simulink model "Test_Arithmetic_Operation_Bit_Comparator_Less_Than"  (Simulink 8.7)
settings: Solver=ode45  StartTime=0.0  StopTime=len  RelTol=1e-3
libraries: Arithmetic_Operations_Lib x1
settings Model: Creator=uzivatel  LastModifiedBy=Jozko Mrkvicka
settings DebuggingCC: SolverPrmCheckMsg=warning  StateNameClashWarn=warning

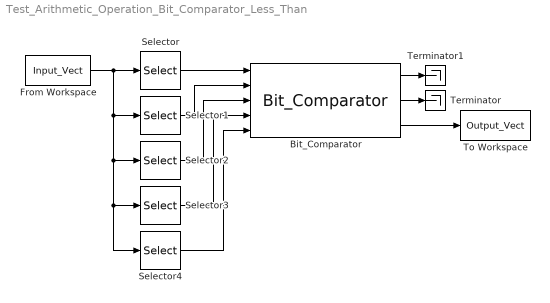
== system Test_Arithmetic_Operation_Bit_Comparator_Less_Than ==
  Bit_Comparator : Arithmetic_Operations_Lib/Arithmetic_Operations_Lib/Bit_Comparator
  From Workspace : FromWorkspace  VariableName=Input_Vect  SampleTime=1  Interpolate=off  OutputAfterFinalValue=Holding final value
  Selector : Selector  IndexMode=Zero-based  InputPortWidth=5  SampleTime=1  IndexOptions=Index vector (dialog)  Indices=0  OutputSizes=1
  Selector1 : Selector  IndexMode=Zero-based  InputPortWidth=5  SampleTime=1  IndexOptions=Index vector (dialog)  Indices=1  OutputSizes=1
  Selector2 : Selector  IndexMode=Zero-based  InputPortWidth=5  SampleTime=1  IndexOptions=Index vector (dialog)  Indices=2  OutputSizes=1
  Selector3 : Selector  IndexMode=Zero-based  InputPortWidth=5  SampleTime=1  IndexOptions=Index vector (dialog)  Indices=3  OutputSizes=1
  Selector4 : Selector  IndexMode=Zero-based  InputPortWidth=5  SampleTime=1  IndexOptions=Index vector (dialog)  Indices=4  OutputSizes=1
  Terminator : Terminator
  Terminator1 : Terminator
  To Workspace : ToWorkspace  VariableName=Output_Vect  SampleTime=1
  wires:
  From Workspace/1 -> Selector4/1, Selector3/1, Selector2/1, Selector1/1, Selector/1
  Selector/1 -> Bit_Comparator/1
  Bit_Comparator/2 -> Terminator/1
  Bit_Comparator/3 -> To Workspace/1
  Selector1/1 -> Bit_Comparator/2
  Selector2/1 -> Bit_Comparator/3
  Selector3/1 -> Bit_Comparator/4
  Selector4/1 -> Bit_Comparator/5
  Bit_Comparator/1 -> Terminator1/1
